simulink model "test_simu3"  (R2019a)
settings: Solver=VariableStepAuto  StartTime=0.0  StopTime=30  RelTol=1e-3
values from neighbouring files (symbols this model uses):
  b = 3.0 *10^-5    (= 3e-05)    [constants_drone.m]    (also in drone.m)
  d = 1.1*10^-6    (= 1.1e-06)    [constants_drone.m]    (also in drone.m)
  Ixx = 0.0196    [constants_drone.m]
  Iyy = Ixx    (= 0.0196)    [constants_drone.m]
  Izz = 0.0264    [constants_drone.m]
  Jr = (1/2)*(m*0.01^2)    (= 1.25e-05)    [constants_drone.m]    (also in drone.m = 0.001)
  l = 0.25    [constants_drone.m]    (also in drone.m)
  m = 0.25    [constants_drone.m]    (also in drone.m = 0.5; drone_test.m)
  omega1 = 475    [constants_drone.m]
  omega2 = 500    [constants_drone.m]
  omega3 = 475    [constants_drone.m]
  omega4 = 475    [constants_drone.m]
undefined symbols (not defined in the file or in its folder): magnitude
settings Model: Creator=Emil  LastModifiedBy=Emil

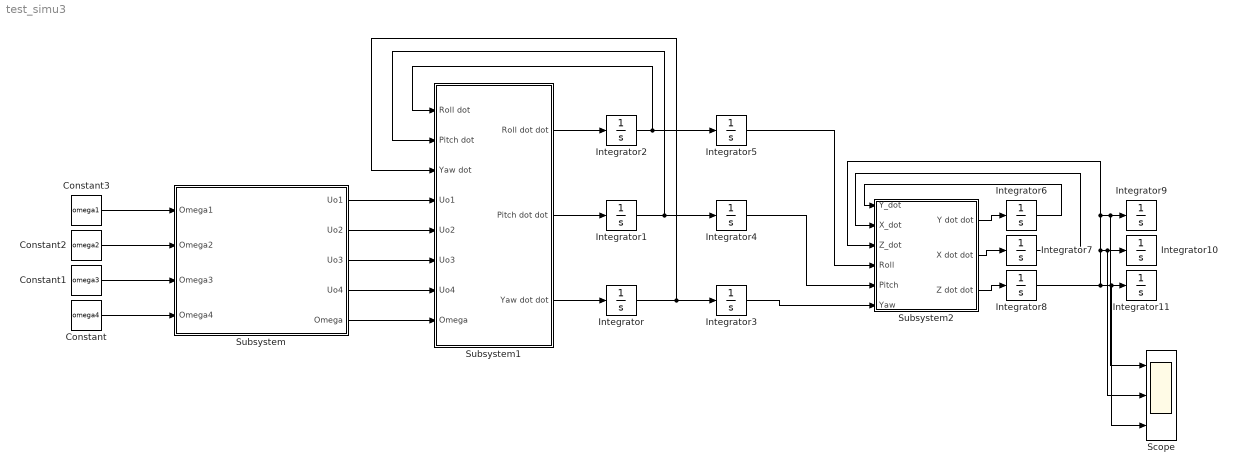
== system test_simu3 ==
  Constant : Constant  Value=omega4
  Constant1 : Constant  Value=omega3
  Constant2 : Constant  Value=omega2
  Constant3 : Constant  Value=omega1
  Integrator{,1..11} (12 alike) : Integrator
  Scope : Scope  NumInputPorts=3
  Subsystem : Subsystem
  Subsystem1 : Subsystem
  Subsystem2 : Subsystem
  wires:
  Constant3/1 -> Subsystem/1(Omega1)
  Constant2/1 -> Subsystem/2(Omega2)
  Constant1/1 -> Subsystem/3(Omega3)
  Constant/1 -> Subsystem/4(Omega4)
  Subsystem/1(Uo1) -> Subsystem1/4(Uo1)
  Subsystem/2(Uo2) -> Subsystem1/5(Uo2)
  Subsystem/3(Uo3) -> Subsystem1/6(Uo3)
  Subsystem/4(Uo4) -> Subsystem1/7(Uo4)
  Subsystem/5(Omega) -> Subsystem1/8(Omega)
  Subsystem1/1(Roll dot dot) -> Integrator2/1
  Subsystem1/2(Pitch dot dot) -> Integrator1/1
  Subsystem1/3(Yaw dot dot) -> Integrator/1
  Integrator/1 -> Integrator3/1, Subsystem1/3(Yaw dot)
  Integrator1/1 -> Integrator4/1, Subsystem1/2(Pitch dot)
  Integrator2/1 -> Integrator5/1, Subsystem1/1(Roll dot)
  Integrator5/1 -> Subsystem2/4(Roll)
  Integrator4/1 -> Subsystem2/5(Pitch)
  Integrator3/1 -> Subsystem2/6(Yaw)
  Subsystem2/1(Y dot dot) -> Integrator6/1
  Subsystem2/2(X dot dot) -> Integrator7/1
  Subsystem2/3(Z dot dot) -> Integrator8/1
  Integrator6/1 -> Subsystem2/1(Y_dot)
  Integrator7/1 -> Subsystem2/2(X_dot)
  Integrator8/1 -> Scope/3, Integrator11/1, Scope/2, Integrator10/1, Scope/1, Integrator9/1, Subsystem2/3(Z_dot)

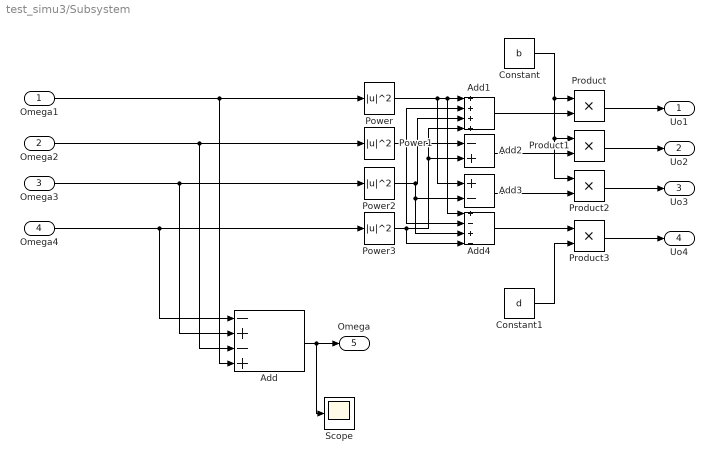
== system test_simu3/Subsystem ==
  Omega1 : Inport
  Omega2 : Inport  Port=2
  Omega3 : Inport  Port=3
  Omega4 : Inport  Port=4
  Add : Sum  Inputs=-+-+
  Add1 : Sum  Inputs=++++
  Add2 : Sum  Inputs=-+
  Add3 : Sum  Inputs=+-
  Add4 : Sum  Inputs=+-+-
  Constant : Constant  Value=b
  Constant1 : Constant  Value=d
  Power{,1..3} (4 alike) : Math  Operator=magnitude^2  SaturateOnIntegerOverflow=on
  Product{,1..3} (4 alike) : Product
  Scope : Scope
  Uo1 : Outport
  Uo2 : Outport  Port=2
  Uo3 : Outport  Port=3
  Uo4 : Outport  Port=4
  Omega : Outport  Port=5
  wires:
  Add4/1 -> Product3/1
  Power3/1 -> Add4/4, Add2/2, Add1/4
  Omega4/1 -> Add/1, Power3/1
  Omega2/1 -> Add/3, Power1/1
  Omega1/1 -> Add/4, Power/1
  Power/1 -> Add3/1, Add4/1, Add1/1
  Omega3/1 -> Add/2, Power2/1
  Constant/1 -> Product2/1, Product1/1, Product/1
  Add2/1 -> Product1/2
  Constant1/1 -> Product3/2
  Product3/1 -> Uo4/1
  Product2/1 -> Uo3/1
  Power1/1 -> Add4/2, Add2/1, Add1/2
  Product1/1 -> Uo2/1
  Add3/1 -> Product2/2
  Power2/1 -> Add4/3, Add3/2, Add1/3
  Add1/1 -> Product/2
  Product/1 -> Uo1/1
  Add/1 -> Scope/1, Omega/1

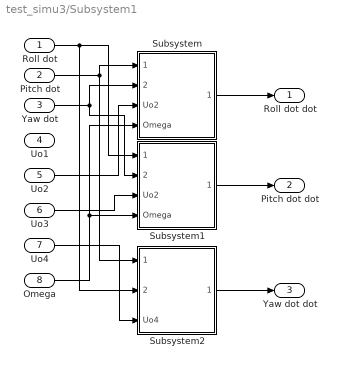
== system test_simu3/Subsystem1 ==
  Roll dot : Inport
  Pitch dot : Inport  Port=2
  Yaw dot : Inport  Port=3
  Uo1 : Inport  Port=4
  Uo2 : Inport  Port=5
  Uo3 : Inport  Port=6
  Uo4 : Inport  Port=7
  Omega : Inport  Port=8
  Subsystem : Subsystem
  Subsystem1 : Subsystem
  Subsystem2 : Subsystem
  Roll dot dot : Outport
  Pitch dot dot : Outport  Port=2
  Yaw dot dot : Outport  Port=3
  wires:
  Pitch dot/1 -> Subsystem2/1(Pitch dot), Subsystem/1(Pitch dot)
  Yaw dot/1 -> Subsystem1/2(Yaw dot), Subsystem/2(Yaw dot)
  Uo2/1 -> Subsystem/3(Uo2)
  Omega/1 -> Subsystem1/4(Omega), Subsystem/4(Omega)
  Subsystem/1(Roll dot dot) -> Roll dot dot/1
  Roll dot/1 -> Subsystem2/2(Roll dot), Subsystem1/1(Roll dot)
  Uo3/1 -> Subsystem1/3(Uo2)
  Subsystem2/1(Yaw dot dot) -> Yaw dot dot/1
  Subsystem1/1(Roll dot dot) -> Pitch dot dot/1
  Uo4/1 -> Subsystem2/3(Uo4)

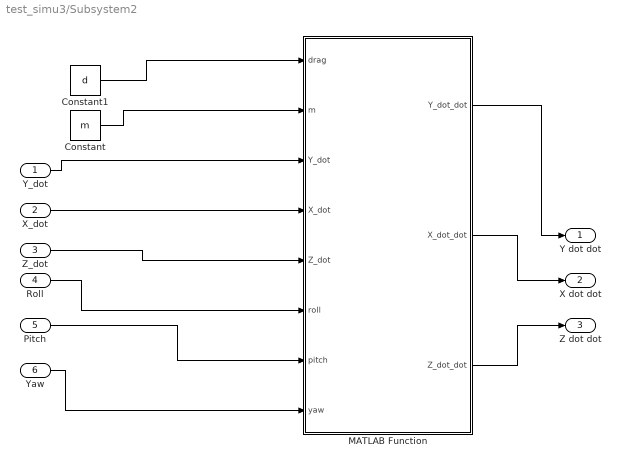
== system test_simu3/Subsystem2 ==
  Y_dot : Inport
  X_dot : Inport  Port=2
  Z_dot : Inport  Port=3
  Roll : Inport  Port=4
  Pitch : Inport  Port=5
  Yaw : Inport  Port=6
  Constant : Constant  Value=m
  Constant1 : Constant  Value=d
  MATLAB Function : MATLAB Function  TreatAsAtomicUnit=on
  Y dot dot : Outport
  X dot dot : Outport  Port=2
  Z dot dot : Outport  Port=3
  wires:
  Roll/1 -> MATLAB Function/6(roll)
  MATLAB Function/1(Y_dot_dot) -> Y dot dot/1
  Pitch/1 -> MATLAB Function/7(pitch)
  Yaw/1 -> MATLAB Function/8(yaw)
  MATLAB Function/2(X_dot_dot) -> X dot dot/1
  MATLAB Function/3(Z_dot_dot) -> Z dot dot/1
  Constant/1 -> MATLAB Function/2(m)
  Constant1/1 -> MATLAB Function/1(drag)
  Y_dot/1 -> MATLAB Function/3(Y_dot)
  X_dot/1 -> MATLAB Function/4(X_dot)
  Z_dot/1 -> MATLAB Function/5(Z_dot)

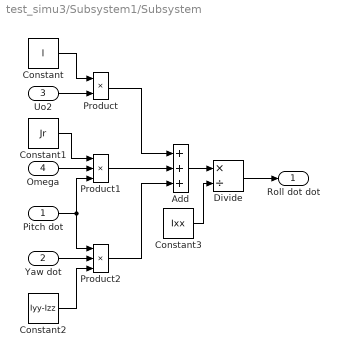
== system test_simu3/Subsystem1/Subsystem ==
  Pitch dot : Inport
  Yaw dot : Inport  Port=2
  Uo2 : Inport  Port=3
  Omega : Inport  Port=4
  Add : Sum  Inputs=+++
  Constant : Constant  Value=l
  Constant1 : Constant  Value=Jr
  Constant2 : Constant  Value=Iyy-Izz
  Constant3 : Constant  Value=Ixx
  Divide : Product  Inputs=*/
  Product : Product
  Product1 : Product  Inputs=3
  Product2 : Product  Inputs=3
  Roll dot dot : Outport
  wires:
  Constant/1 -> Product/1
  Uo2/1 -> Product/2
  Constant1/1 -> Product1/1
  Omega/1 -> Product1/2
  Pitch dot/1 -> Product2/1, Product1/3
  Yaw dot/1 -> Product2/2
  Constant2/1 -> Product2/3
  Product/1 -> Add/1
  Product1/1 -> Add/2
  Product2/1 -> Add/3
  Add/1 -> Divide/1
  Constant3/1 -> Divide/2
  Divide/1 -> Roll dot dot/1

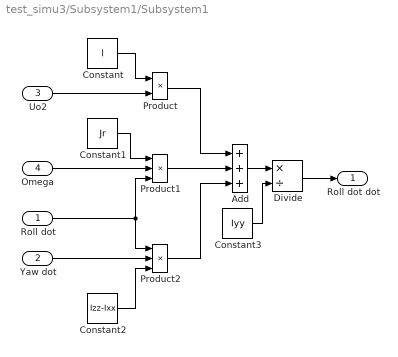
== system test_simu3/Subsystem1/Subsystem1 ==
  Roll dot : Inport
  Yaw dot : Inport  Port=2
  Uo2 : Inport  Port=3
  Omega : Inport  Port=4
  Add : Sum  Inputs=+++
  Constant : Constant  Value=l
  Constant1 : Constant  Value=Jr
  Constant2 : Constant  Value=Izz-Ixx
  Constant3 : Constant  Value=Iyy
  Divide : Product  Inputs=*/
  Product : Product
  Product1 : Product  Inputs=3
  Product2 : Product  Inputs=3
  Roll dot dot : Outport
  wires:
  Divide/1 -> Roll dot dot/1
  Yaw dot/1 -> Product2/2
  Constant3/1 -> Divide/2
  Constant/1 -> Product/1
  Product/1 -> Add/1
  Omega/1 -> Product1/2
  Constant2/1 -> Product2/3
  Add/1 -> Divide/1
  Roll dot/1 -> Product2/1, Product1/3
  Constant1/1 -> Product1/1
  Product2/1 -> Add/3
  Product1/1 -> Add/2
  Uo2/1 -> Product/2

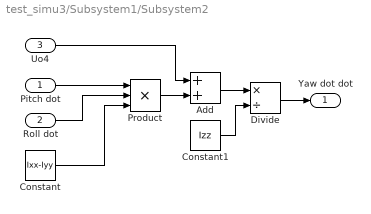
== system test_simu3/Subsystem1/Subsystem2 ==
  Pitch dot : Inport
  Roll dot : Inport  Port=2
  Uo4 : Inport  Port=3
  Add : Sum
  Constant : Constant  Value=Ixx-Iyy
  Constant1 : Constant  Value=Izz
  Divide : Product  Inputs=*/
  Product : Product  Inputs=3
  Yaw dot dot : Outport
  wires:
  Uo4/1 -> Add/1
  Pitch dot/1 -> Product/1
  Roll dot/1 -> Product/2
  Constant/1 -> Product/3
  Product/1 -> Add/2
  Add/1 -> Divide/1
  Divide/1 -> Yaw dot dot/1
  Constant1/1 -> Divide/2

== matlab function test_simu3/Subsystem2/MATLAB Function ==
  data: drag input; m input; Y_dot input; X_dot input; Z_dot input; roll input; Y_dot_dot output; pitch input; yaw input; X_dot_dot output; Z_dot_dot output
function [Y_dot_dot,X_dot_dot, Z_dot_dot] = fcn(drag, m, Y_dot, X_dot, Z_dot, roll, pitch, yaw)
Y_dot_dot = ((cos(yaw)*sin(roll)+sin(yaw)*sin(pitch)*cos(roll)))/m;
X_dot_dot = 1;
Z_dot_dot = 2;
